simulink model "five_bar_model_w_g"  (R2018a)
settings: Solver=ode4  StartTime=0.0  StopTime=10.0  FixedStep=1e-4  RelTol=1e-3
values from neighbouring files (symbols this model uses):
  g = -9.80665    [ddyn5.m]    (also in idyn5.m; test_dynamics.m; test_model.m)
  p0 = p(:,1)    [model_parameters_v_1.m]    (also in test_dynamics.m = [x(i);y(i)]; test_kinematics.m = [0; 0.35]; test_model.m = [x0;y0])
  q = [NaN; NaN; NaN; NaN; NaN]    [fkine5.m]    (also in ikine5.m = [q11;q12;q13;q21;q22]; test_model.m = q_mode(:,4))
  q0 = q(:,1)    [model_parameters_v_1.m]    (also in test_dynamics.m = q0(:,4); test_kinematics.m = q0(:,4); test_model.m = q_mode(:,4))
  t0r0 = t0r(:,1)    [model_parameters_v_1.m]    (also in test_model.m = [0;0])
  t0rd0 = t0rd(:,1)    [model_parameters_v_1.m]    (also in test_model.m = [0;0])
  x0 = p(1,1)    [model_parameters_v_1.m]    (also in test_model.m = 0)
  y0 = p(2,1)    [model_parameters_v_1.m]    (also in test_model.m = 0.35)
undefined symbols (not defined in the file or in its folder): X, Y, Z
libraries: sm_lib x25, nesl_utility x7, simulink x1
(part 1 of 2)
settings Model: Creator=jere  LastModifiedBy=jere

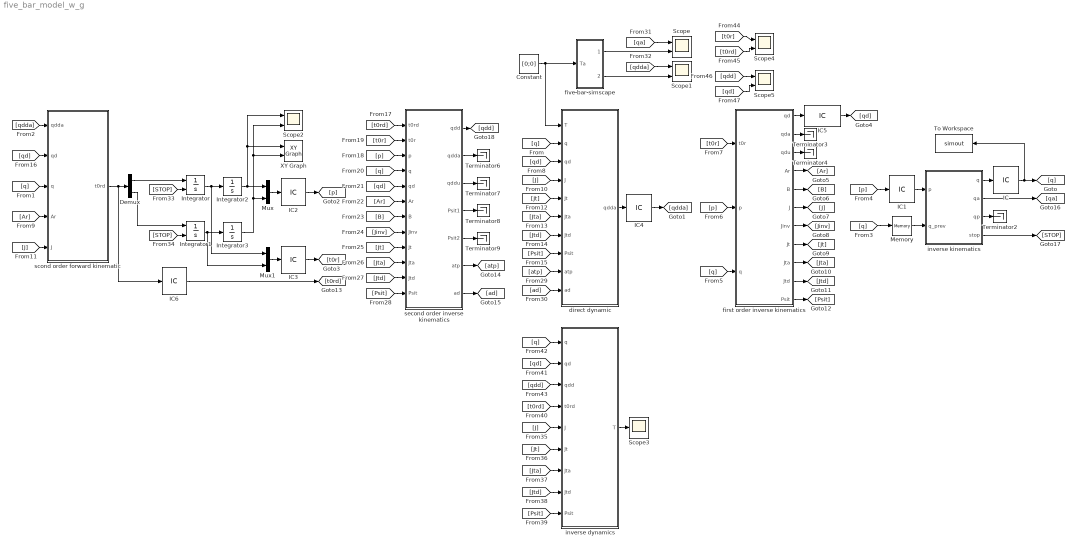
== system five_bar_model_w_g ==
  Constant : Constant  Value=[0;0]
  Demux : Demux  Outputs=2
  IC : InitialCondition  Value=q0
  IC1 : InitialCondition  Value=p0
  IC2 : InitialCondition  Value=p0
  IC3 : InitialCondition  Value=t0r0
  IC4 : InitialCondition  Value=[0;0]
  IC5 : InitialCondition  Value=zeros(5,1)
  IC6 : InitialCondition  Value=t0rd0
  Integrator : Integrator  ExternalReset=level hold
  Integrator1 : Integrator  ExternalReset=level hold
  Integrator2 : Integrator  InitialCondition=x0
  Integrator3 : Integrator  InitialCondition=y0
  Memory : Memory  InitialCondition=q0
  Mux : Mux  Inputs=2
  Mux1 : Mux  Inputs=2
  Scope{,1..2,4..5} (5 alike) : Scope  NumInputPorts=2
  Scope3 : Scope
  Terminator{2..4,6..9} (7 alike) : Terminator
  To Workspace : ToWorkspace  VariableName=simout  SaveFormat=Timeseries  SampleTime=-1
  XY Graph : simulink/Sinks/XY Graph  xmin=-1  xmax=1  ymin=-1  ymax=1  st=-1
  direct dynamic : MATLAB Function  TreatAsAtomicUnit=on
  first order inverse kinematics : MATLAB Function  TreatAsAtomicUnit=on
  five-bar-simscape : Subsystem
  inverse dynamics : MATLAB Function  TreatAsAtomicUnit=on
  inverse kinematics : MATLAB Function  TreatAsAtomicUnit=on
  scond order forward kinematic : MATLAB Function  TreatAsAtomicUnit=on
  second order inverse kinematics : MATLAB Function  TreatAsAtomicUnit=on
  wires:
  Constant/1 -> direct dynamic/1(T), five-bar-simscape/1(Ta)
  five-bar-simscape/2(qdda_o) -> Scope1/2
  [q] -> direct dynamic/2(q)
  [q] -> scond order forward kinematic/3(q)
  IC/1 -> [q], To Workspace/1
  [qdda] -> scond order forward kinematic/1(qdda)
  [q] -> Memory/1
  Memory/1 -> inverse kinematics/2(q_prev)
  inverse kinematics/1(q) -> IC/1
  inverse kinematics/2(qa) -> [qa]
  inverse kinematics/3(qp) -> Terminator2/1
  Integrator/1 -> Integrator2/1, Mux1/1
  Integrator1/1 -> Integrator3/1, Mux1/2
  scond order forward kinematic/1(t0rd) -> Demux/1, IC6/1
  Demux/1 -> Integrator/1
  Demux/2 -> Integrator1/1
  Integrator2/1 -> Scope2/1, XY Graph/1, Mux/1
  Integrator3/1 -> XY Graph/2, Scope2/2, Mux/2
  Mux/1 -> IC2/1
  [p] -> IC1/1
  IC1/1 -> inverse kinematics/1(p)
  [q] -> first order inverse kinematics/3(q)
  [p] -> first order inverse kinematics/2(p)
  [t0r] -> first order inverse kinematics/1(t0r)
  Mux1/1 -> IC3/1
  first order inverse kinematics/1(qd) -> IC5/1
  [qd] -> direct dynamic/3(qd)
  first order inverse kinematics/2(qda) -> Terminator3/1
  first order inverse kinematics/3(qdu) -> Terminator4/1
  first order inverse kinematics/4(Ar) -> [Ar]
  [Ar] -> scond order forward kinematic/4(Ar)
  first order inverse kinematics/5(B) -> [B]
  first order inverse kinematics/6(J) -> [J]
  [J] -> direct dynamic/4(J)
  [J] -> scond order forward kinematic/5(J)
  first order inverse kinematics/7(Jinv) -> [Jinv]
  first order inverse kinematics/8(Jt) -> [Jt]
  [Jt] -> direct dynamic/5(Jt)
  first order inverse kinematics/9(Jta) -> [Jta]
  [Jta] -> direct dynamic/6(Jta)
  first order inverse kinematics/10(Jtd) -> [Jtd]
  [Jtd] -> direct dynamic/7(Jtd)
  first order inverse kinematics/11(Psit) -> [Psit]
  [Psit] -> direct dynamic/8(Psit)
  [qd] -> scond order forward kinematic/2(qd)
  [t0rd] -> second order inverse kinematics/1(t0rd)
  [p] -> second order inverse kinematics/3(p)
  [t0r] -> second order inverse kinematics/2(t0r)
  IC3/1 -> [t0r]
  IC2/1 -> [p]
  [q] -> second order inverse kinematics/4(q)
  [qd] -> second order inverse kinematics/5(qd)
  [Ar] -> second order inverse kinematics/6(Ar)
  [B] -> second order inverse kinematics/7(B)
  [Jinv] -> second order inverse kinematics/8(Jinv)
  [Jt] -> second order inverse kinematics/9(Jt)
  [Jta] -> second order inverse kinematics/10(Jta)
  [Jtd] -> second order inverse kinematics/11(Jtd)
  [Psit] -> second order inverse kinematics/12(Psit)
  second order inverse kinematics/6(atp) -> [atp]
  second order inverse kinematics/7(ad) -> [ad]
  [atp] -> direct dynamic/9(atp)
  [ad] -> direct dynamic/10(ad)
  second order inverse kinematics/1(qdd) -> [qdd]
  second order inverse kinematics/2(qdda) -> Terminator6/1
  second order inverse kinematics/3(qddu) -> Terminator7/1
  second order inverse kinematics/4(Psit1) -> Terminator8/1
  second order inverse kinematics/5(Psit2) -> Terminator9/1
  five-bar-simscape/1(qa_o) -> Scope/2
  direct dynamic/1(qdda) -> IC4/1
  IC5/1 -> [qd]
  [qa] -> Scope/1
  [qdda] -> Scope1/1
  inverse kinematics/4(stop) -> [STOP]
  [STOP] -> Integrator/2
  [STOP] -> Integrator1/2
  inverse dynamics/1(T) -> Scope3/1
  [J] -> inverse dynamics/5(J)
  [Jt] -> inverse dynamics/6(Jt)
  [Jta] -> inverse dynamics/7(Jta)
  [Jtd] -> inverse dynamics/8(Jtd)
  [Psit] -> inverse dynamics/9(Psit)
  [t0rd] -> inverse dynamics/4(t0rd)
  [qd] -> inverse dynamics/2(qd)
  [q] -> inverse dynamics/1(q)
  [qdd] -> inverse dynamics/3(qdd)
  [t0r] -> Scope4/1
  [t0rd] -> Scope4/2
  [qdd] -> Scope5/1
  [qd] -> Scope5/2
  IC4/1 -> [qdda]
  IC6/1 -> [t0rd]

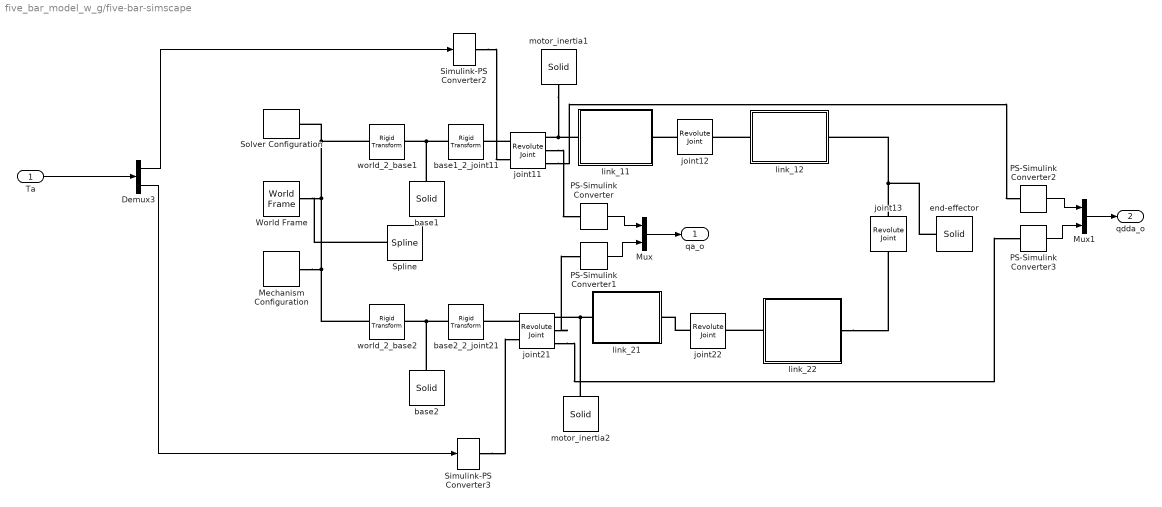
== system five_bar_model_w_g/five-bar-simscape ==
  Ta : Inport
  Demux3 : Demux  Outputs=2
  Mechanism Configuration : sm_lib/Utilities/Mechanism Configuration  UniformGravity=Constant  GravityVector=[0 -9.80665 0]  GravityUnits=m/s^2  LinearizationDelta=0.001
  Mux : Mux  Inputs=2
  Mux1 : Mux  Inputs=2
  PS-Simulink Converter : nesl_utility/PS-Simulink Converter  PhysicalDomain=network_engine_domain  SubClassName=ps_output  LeftPortType=input  RightPortType=output  PseudoPeriodic=off  Frequencies=[]  Unit=rad  AffineConversion=off
  PS-Simulink Converter1 : nesl_utility/PS-Simulink Converter  PhysicalDomain=network_engine_domain  SubClassName=ps_output  LeftPortType=input  RightPortType=output  PseudoPeriodic=off  Frequencies=[]  Unit=rad  AffineConversion=off
  PS-Simulink Converter2 : nesl_utility/PS-Simulink Converter  PhysicalDomain=network_engine_domain  SubClassName=ps_output  LeftPortType=input  RightPortType=output  PseudoPeriodic=off  Frequencies=[]  Unit=1  AffineConversion=off
  PS-Simulink Converter3 : nesl_utility/PS-Simulink Converter  PhysicalDomain=network_engine_domain  SubClassName=ps_output  LeftPortType=input  RightPortType=output  PseudoPeriodic=off  Frequencies=[]  Unit=1  AffineConversion=off
  Simulink-PS Converter2 : nesl_utility/Simulink-PS Converter  PhysicalDomain=network_engine_domain  SubClassName=ps_input  LeftPortType=input  RightPortType=output  PseudoPeriodic=off  Frequencies=[]  NoiseDistribution=none  NoiseParameters=[]  Unit=N*m  AffineConversion=off  FilteringAndDerivatives=provide  SimscapeFilterOrder=1  InputFilterTimeConstant=0.001  UdotUserProvided=0
  Simulink-PS Converter3 : nesl_utility/Simulink-PS Converter  PhysicalDomain=network_engine_domain  SubClassName=ps_input  LeftPortType=input  RightPortType=output  PseudoPeriodic=off  Frequencies=[]  NoiseDistribution=none  NoiseParameters=[]  Unit=N*m  AffineConversion=off  FilteringAndDerivatives=provide  SimscapeFilterOrder=1  InputFilterTimeConstant=0.001  UdotUserProvided=0
  Solver Configuration : nesl_utility/Solver Configuration  PhysicalDomain=network_engine_domain  SubClassName=solver  LeftPortType=input  RightPortType=generic  Tones=[]  Harmonics=[]  SimulateNoise=off  Profile=off  UseLocalSampling=off  EnableSwitchedLinearOptims=on  FrequencyDomain=off  UseCCode=off  RelTol=0.001  AbsTol=1e-06  MinStep=1e-09  ToWorkspace=off  RevertToSquareIcSolve=off  NumHomotopyIterations=100  PhasorMode=off  PhasorModeNumHarmonics=1  DoDC=off  ResidualTolerance=1e-09  UseLocalSolver=off  LocalSolverChoice=NE_BACKWARD_EULER_ADVANCER  LocalSolverSampleTime=0.001  DoFixedCost=off  MaxNonlinIter=3  MaxModeIter=2  LinearAlgebra=Sparse  EquationFormulation=NE_TIME_EF  DelaysMemoryBudget=1024  AutomaticFiltering=on  FilteringTimeConstant=0.001
  Spline : sm_lib/Curves and Surfaces/Spline  DataPoints=[-0.1 0.3; 0.1 0.3]  DataPointsUnits=m  EndConditionType=Natural  GraphicType=FromGeometry  MarkerShape=Sphere  MarkerSize=10  GraphicVisPropType=SimpleVisualProperties  GraphicDiffuseColor=[0 0 0]  GraphicSpecularColor=[0.5 0.5 0.5 1.0]  GraphicAmbientColor=[0.15 0.15 0.15 1.0]  GraphicEmissiveColor=[0.0 0.0 0.0 1.0]  GraphicShininess=75  GraphicOpacity=1.0
      settings: SourceProductName=Simscape Multibody
  World Frame : sm_lib/Frames and Transforms/World Frame
  base1 : sm_lib/Body Elements/Solid  InertiaType=PointMass  Mass=1.72  MassUnits=kg  CenterOfMass=[0 0 0]  CenterOfMassUnits=m  MomentsOfInertia=[1 1 1]  MomentsOfInertiaUnits=kg*m^2  ProductsOfInertia=[0 0 0]  ProductsOfInertiaUnits=kg*m^2  DensityBased=on  Density=1000  DensityUnits=kg/m^3  DoExposeReferenceFrame=on  SerializedFrames=<Frames/>  GraphicType=FromGeometry  MarkerShape=Sphere  MarkerSize=10  GraphicVisPropType=SimpleVisualProperties  GraphicDiffuseColor=[1.0 1.0 0.0]  GraphicSpecularColor=[0.5 0.5 0.5 1.0]  GraphicAmbientColor=[0.15 0.15 0.15 1.0]  GraphicEmissiveColor=[0.0 0.0 0.0 1.0]  GraphicShininess=75  GraphicOpacity=1.0  GeometryShape=FromFile  RectangleSize=[1 1]  RectangleSizeUnits=m  BrickDimensions=[1 1 1]  BrickDimensionUnits=m  CylinderRadius=1  CylinderRadiusUnits=m  CylinderLength=1  CylinderLengthUnits=m  SphereRadius=1  SphereRadiusUnits=m  EllipsoidRadii=[1 1 1]  EllipsoidRadiiUnits=m  ExtrusionCrossSection=[1 1; -1 1; -1 -1; 1 -1]  ExtrusionCrossSectionUnits=m  ExtrusionLength=1  ExtrusionLengthUnits=m  PolygonNumSides=3  PolygonOuterRadius=1  PolygonOuterRadiusUnits=m  ExtGeomFileType=STL  ExtGeomFileName=/home/jere/Documentos/simulacionPF/5-bar-model/meshes/nema23_75mm_8mm.stl  ExtGeomFileUnits=mm  RevolutionCrossSection=[1 1; 1 -1; 2 -1; 2 1]  RevolutionCrossSectionUnits=m  RevolutionExtent=Full  RevolutionAngle=180  RevolutionAngleUnits=deg
  base1_2_joint11 : sm_lib/Frames and Transforms/Rigid Transform  TranslationMethod=Cartesian  TranslationStandardOffset=0  TranslationLengthUnit=mm  TranslationStandardAxis=+Z  TranslationCartesianOffset=[0 0 2]  TranslationROffset=0  TranslationROffsetUnits=m  TranslationZOffset=0  TranslationZOffsetUnits=m  TranslationThetaOffset=0  TranslationThetaOffsetUnits=deg  RotationMethod=None  RotationAngleUnits=deg  RotationStandardAxis=+Z  RotationAngle=0.0  RotationArbitraryAxis=[0 0 1]  FollAlignAxisA=+X  BaseAlignAxisA=+Y  FollAlignAxisB=+Y  BaseAlignAxisB=+Z  RotationSequenceAxes=FollowerAxes  RotationSequence=XYX  RotationSequenceAngles=[0 0 0]  RotationSequenceAnglesUnits=deg  RotationMatrix=[1 0 0; 0 1 0; 0 0 1]
  base2 : sm_lib/Body Elements/Solid  InertiaType=PointMass  Mass=1.72  MassUnits=kg  CenterOfMass=[0 0 0]  CenterOfMassUnits=m  MomentsOfInertia=[1 1 1]  MomentsOfInertiaUnits=kg*m^2  ProductsOfInertia=[0 0 0]  ProductsOfInertiaUnits=kg*m^2  DensityBased=on  Density=1000  DensityUnits=kg/m^3  DoExposeReferenceFrame=on  SerializedFrames=<Frames/>  GraphicType=FromGeometry  MarkerShape=Sphere  MarkerSize=10  GraphicVisPropType=SimpleVisualProperties  GraphicDiffuseColor=[1.0 1.0 0.0]  GraphicSpecularColor=[0.5 0.5 0.5 1.0]  GraphicAmbientColor=[0.15 0.15 0.15 1.0]  GraphicEmissiveColor=[0.0 0.0 0.0 1.0]  GraphicShininess=75  GraphicOpacity=1.0  GeometryShape=FromFile  RectangleSize=[1 1]  RectangleSizeUnits=m  BrickDimensions=[1 1 1]  BrickDimensionUnits=m  CylinderRadius=1  CylinderRadiusUnits=m  CylinderLength=1  CylinderLengthUnits=m  SphereRadius=1  SphereRadiusUnits=m  EllipsoidRadii=[1 1 1]  EllipsoidRadiiUnits=m  ExtrusionCrossSection=[1 1; -1 1; -1 -1; 1 -1]  ExtrusionCrossSectionUnits=m  ExtrusionLength=1  ExtrusionLengthUnits=m  PolygonNumSides=3  PolygonOuterRadius=1  PolygonOuterRadiusUnits=m  ExtGeomFileType=STL  ExtGeomFileName=/home/jere/Documentos/simulacionPF/5-bar-model/meshes/nema23_75mm_8mm.stl  ExtGeomFileUnits=mm  RevolutionCrossSection=[1 1; 1 -1; 2 -1; 2 1]  RevolutionCrossSectionUnits=m  RevolutionExtent=Full  RevolutionAngle=180  RevolutionAngleUnits=deg
  base2_2_joint21 : sm_lib/Frames and Transforms/Rigid Transform  TranslationMethod=Cartesian  TranslationStandardOffset=0  TranslationLengthUnit=mm  TranslationStandardAxis=+Z  TranslationCartesianOffset=[0 0 2]  TranslationROffset=0  TranslationROffsetUnits=m  TranslationZOffset=0  TranslationZOffsetUnits=m  TranslationThetaOffset=0  TranslationThetaOffsetUnits=deg  RotationMethod=None  RotationAngleUnits=deg  RotationStandardAxis=+Z  RotationAngle=0.0  RotationArbitraryAxis=[0 0 1]  FollAlignAxisA=+X  BaseAlignAxisA=+Y  FollAlignAxisB=+Y  BaseAlignAxisB=+Z  RotationSequenceAxes=FollowerAxes  RotationSequence=XYX  RotationSequenceAngles=[0 0 0]  RotationSequenceAnglesUnits=deg  RotationMatrix=[1 0 0; 0 1 0; 0 0 1]
  end-effector : sm_lib/Body Elements/Solid  InertiaType=PointMass  Mass=0.272  MassUnits=kg  CenterOfMass=[0 0 0]  CenterOfMassUnits=m  MomentsOfInertia=[1 1 1]  MomentsOfInertiaUnits=kg*m^2  ProductsOfInertia=[0 0 0]  ProductsOfInertiaUnits=kg*m^2  DensityBased=on  Density=1000  DensityUnits=kg/m^3  DoExposeReferenceFrame=on  SerializedFrames=<Frames/>  GraphicType=FromGeometry  MarkerShape=Sphere  MarkerSize=10  GraphicVisPropType=SimpleVisualProperties  GraphicDiffuseColor=[1.0 1.0 0.0]  GraphicSpecularColor=[0.5 0.5 0.5 1.0]  GraphicAmbientColor=[0.15 0.15 0.15 1.0]  GraphicEmissiveColor=[0.0 0.0 0.0 1.0]  GraphicShininess=75  GraphicOpacity=1.0  GeometryShape=Sphere  RectangleSize=[1 1]  RectangleSizeUnits=m  BrickDimensions=[1 1 1]  BrickDimensionUnits=m  CylinderRadius=1  CylinderRadiusUnits=m  CylinderLength=1  CylinderLengthUnits=m  SphereRadius=1  SphereRadiusUnits=mm  EllipsoidRadii=[1 1 1]  EllipsoidRadiiUnits=m  ExtrusionCrossSection=[1 1; -1 1; -1 -1; 1 -1]  ExtrusionCrossSectionUnits=m  ExtrusionLength=1  ExtrusionLengthUnits=m  PolygonNumSides=3  PolygonOuterRadius=1  PolygonOuterRadiusUnits=m  ExtGeomFileType=STL  ExtGeomFileName=D:\PartsMechanism\propiedades\nema23_75mm_8mm.stl  ExtGeomFileUnits=mm  RevolutionCrossSection=[1 1; 1 -1; 2 -1; 2 1]  RevolutionCrossSectionUnits=m  RevolutionExtent=Full  RevolutionAngle=180  RevolutionAngleUnits=deg
  joint11 : sm_lib/Joints/Revolute Joint  SenseConstraintForce=off  SenseConstraintForceX=off  SenseConstraintForceY=off  SenseConstraintForceZ=off  SenseConstraintTorque=off  SenseConstraintTorqueX=off  SenseConstraintTorqueY=off  SenseConstraintTorqueZ=off  SenseTotalForce=off  SenseTotalForceX=off  SenseTotalForceY=off  SenseTotalForceZ=off  SenseTotalTorque=off  SenseTotalTorqueX=off  SenseTotalTorqueY=off  SenseTotalTorqueZ=off  CompositeWrenchDir=FollowerOnBase  CompositeWrenchFrame=BaseFrame  EquilibriumPosition=0  EquilibriumPositionUnits=rad  SpringStiffness=0  SpringStiffnessUnits=N*m/deg  DampingCoefficient=1.5e-1  DampingCoefficientUnits=N*m/(rad/s)  TorqueActuationMode=InputTorque  MotionActuationMode=ComputedMotion  SensePosition=on  SenseVelocity=off  SenseAcceleration=on  SenseTorqueForce=off  PositionTargetSpecify=on  PositionTargetPriority=High  PositionTargetValue=q(1,1)  PositionTargetValueUnits=rad  VelocityTargetSpecify=off  VelocityTargetPriority=High  VelocityTargetValue=1  VelocityTargetValueUnits=rad/s
  joint12 : sm_lib/Joints/Revolute Joint  SenseConstraintForce=off  SenseConstraintForceX=off  SenseConstraintForceY=off  SenseConstraintForceZ=off  SenseConstraintTorque=off  SenseConstraintTorqueX=off  SenseConstraintTorqueY=off  SenseConstraintTorqueZ=off  SenseTotalForce=off  SenseTotalForceX=off  SenseTotalForceY=off  SenseTotalForceZ=off  SenseTotalTorque=off  SenseTotalTorqueX=off  SenseTotalTorqueY=off  SenseTotalTorqueZ=off  CompositeWrenchDir=FollowerOnBase  CompositeWrenchFrame=BaseFrame  EquilibriumPosition=0  EquilibriumPositionUnits=rad  SpringStiffness=0  SpringStiffnessUnits=N*m/deg  DampingCoefficient=0  DampingCoefficientUnits=N*m/(rad/s)  TorqueActuationMode=NoTorque  MotionActuationMode=ComputedMotion  SensePosition=off  SenseVelocity=off  SenseAcceleration=off  SenseTorqueForce=off  PositionTargetSpecify=off  PositionTargetPriority=High  PositionTargetValue=q(2,1)  PositionTargetValueUnits=rad  VelocityTargetSpecify=off  VelocityTargetPriority=High  VelocityTargetValue=100  VelocityTargetValueUnits=rad/s
  joint13 : sm_lib/Joints/Revolute Joint  SenseConstraintForce=off  SenseConstraintForceX=off  SenseConstraintForceY=off  SenseConstraintForceZ=off  SenseConstraintTorque=off  SenseConstraintTorqueX=off  SenseConstraintTorqueY=off  SenseConstraintTorqueZ=off  SenseTotalForce=off  SenseTotalForceX=off  SenseTotalForceY=off  SenseTotalForceZ=off  SenseTotalTorque=off  SenseTotalTorqueX=off  SenseTotalTorqueY=off  SenseTotalTorqueZ=off  CompositeWrenchDir=FollowerOnBase  CompositeWrenchFrame=BaseFrame  EquilibriumPosition=0  EquilibriumPositionUnits=rad  SpringStiffness=0  SpringStiffnessUnits=N*m/deg  DampingCoefficient=0  DampingCoefficientUnits=N*m/(rad/s)  TorqueActuationMode=NoTorque  MotionActuationMode=ComputedMotion  SensePosition=off  SenseVelocity=off  SenseAcceleration=off  SenseTorqueForce=off  PositionTargetSpecify=off  PositionTargetPriority=High  PositionTargetValue=270  PositionTargetValueUnits=rad  VelocityTargetSpecify=off  VelocityTargetPriority=High  VelocityTargetValue=100  VelocityTargetValueUnits=rad/s
  joint21 : sm_lib/Joints/Revolute Joint  SenseConstraintForce=off  SenseConstraintForceX=off  SenseConstraintForceY=off  SenseConstraintForceZ=off  SenseConstraintTorque=off  SenseConstraintTorqueX=off  SenseConstraintTorqueY=off  SenseConstraintTorqueZ=off  SenseTotalForce=off  SenseTotalForceX=off  SenseTotalForceY=off  SenseTotalForceZ=off  SenseTotalTorque=off  SenseTotalTorqueX=off  SenseTotalTorqueY=off  SenseTotalTorqueZ=off  CompositeWrenchDir=FollowerOnBase  CompositeWrenchFrame=BaseFrame  EquilibriumPosition=0  EquilibriumPositionUnits=rad  SpringStiffness=0  SpringStiffnessUnits=N*m/deg  DampingCoefficient=1.5e-1  DampingCoefficientUnits=N*m/(rad/s)  TorqueActuationMode=InputTorque  MotionActuationMode=ComputedMotion  SensePosition=on  SenseVelocity=off  SenseAcceleration=on  SenseTorqueForce=off  PositionTargetSpecify=on  PositionTargetPriority=High  PositionTargetValue=q(4,1)  PositionTargetValueUnits=rad  VelocityTargetSpecify=off  VelocityTargetPriority=High  VelocityTargetValue=100  VelocityTargetValueUnits=rad/s
  joint22 : sm_lib/Joints/Revolute Joint  SenseConstraintForce=off  SenseConstraintForceX=off  SenseConstraintForceY=off  SenseConstraintForceZ=off  SenseConstraintTorque=off  SenseConstraintTorqueX=off  SenseConstraintTorqueY=off  SenseConstraintTorqueZ=off  SenseTotalForce=off  SenseTotalForceX=off  SenseTotalForceY=off  SenseTotalForceZ=off  SenseTotalTorque=off  SenseTotalTorqueX=off  SenseTotalTorqueY=off  SenseTotalTorqueZ=off  CompositeWrenchDir=FollowerOnBase  CompositeWrenchFrame=BaseFrame  EquilibriumPosition=0  EquilibriumPositionUnits=rad  SpringStiffness=0  SpringStiffnessUnits=N*m/deg  DampingCoefficient=0  DampingCoefficientUnits=N*m/(rad/s)  TorqueActuationMode=NoTorque  MotionActuationMode=ComputedMotion  SensePosition=off  SenseVelocity=off  SenseAcceleration=off  SenseTorqueForce=off  PositionTargetSpecify=off  PositionTargetPriority=High  PositionTargetValue=q(5,1)  PositionTargetValueUnits=rad  VelocityTargetSpecify=off  VelocityTargetPriority=High  VelocityTargetValue=100  VelocityTargetValueUnits=rad/s
  link_11 : Subsystem
  link_12 : Subsystem
  link_21 : Subsystem
  link_22 : Subsystem
  motor_inertia1 : sm_lib/Body Elements/Solid  InertiaType=Custom  Mass=0  MassUnits=kg  CenterOfMass=[0 0 0]  CenterOfMassUnits=m  MomentsOfInertia="[0  0 4.8e-5]"  MomentsOfInertiaUnits=kg*m^2  ProductsOfInertia=[0 0 0]  ProductsOfInertiaUnits=kg*m^2  DensityBased=on  Density=1000  DensityUnits=kg/m^3  DoExposeReferenceFrame=on  SerializedFrames=<Frames/>  GraphicType=FromGeometry  MarkerShape=Sphere  MarkerSize=10  GraphicVisPropType=SimpleVisualProperties  GraphicDiffuseColor=[1.0 1.0 0.0]  GraphicSpecularColor=[0.5 0.5 0.5 1.0]  GraphicAmbientColor=[0.15 0.15 0.15 1.0]  GraphicEmissiveColor=[0.0 0.0 0.0 1.0]  GraphicShininess=75  GraphicOpacity=1.0  GeometryShape=Sphere  RectangleSize=[1 1]  RectangleSizeUnits=m  BrickDimensions=[1 1 1]  BrickDimensionUnits=m  CylinderRadius=1  CylinderRadiusUnits=m  CylinderLength=1  CylinderLengthUnits=m  SphereRadius=1  SphereRadiusUnits=mm  EllipsoidRadii=[1 1 1]  EllipsoidRadiiUnits=m  ExtrusionCrossSection=[1 1; -1 1; -1 -1; 1 -1]  ExtrusionCrossSectionUnits=m  ExtrusionLength=1  ExtrusionLengthUnits=m  PolygonNumSides=3  PolygonOuterRadius=1  PolygonOuterRadiusUnits=m  ExtGeomFileType=STL  ExtGeomFileName=D:\PartsMechanism\propiedades\nema23_75mm_8mm.stl  ExtGeomFileUnits=mm  RevolutionCrossSection=[1 1; 1 -1; 2 -1; 2 1]  RevolutionCrossSectionUnits=m  RevolutionExtent=Full  RevolutionAngle=180  RevolutionAngleUnits=deg
  motor_inertia2 : sm_lib/Body Elements/Solid  InertiaType=Custom  Mass=0  MassUnits=kg  CenterOfMass=[0 0 0]  CenterOfMassUnits=m  MomentsOfInertia=[0 0 4.8e-5]  MomentsOfInertiaUnits=kg*m^2  ProductsOfInertia=[0 0 0]  ProductsOfInertiaUnits=kg*m^2  DensityBased=on  Density=1000  DensityUnits=kg/m^3  DoExposeReferenceFrame=on  SerializedFrames=<Frames/>  GraphicType=FromGeometry  MarkerShape=Sphere  MarkerSize=10  GraphicVisPropType=SimpleVisualProperties  GraphicDiffuseColor=[1.0 1.0 0.0]  GraphicSpecularColor=[0.5 0.5 0.5 1.0]  GraphicAmbientColor=[0.15 0.15 0.15 1.0]  GraphicEmissiveColor=[0.0 0.0 0.0 1.0]  GraphicShininess=75  GraphicOpacity=1.0  GeometryShape=Sphere  RectangleSize=[1 1]  RectangleSizeUnits=m  BrickDimensions=[1 1 1]  BrickDimensionUnits=m  CylinderRadius=1  CylinderRadiusUnits=m  CylinderLength=1  CylinderLengthUnits=m  SphereRadius=1  SphereRadiusUnits=mm  EllipsoidRadii=[1 1 1]  EllipsoidRadiiUnits=m  ExtrusionCrossSection=[1 1; -1 1; -1 -1; 1 -1]  ExtrusionCrossSectionUnits=m  ExtrusionLength=1  ExtrusionLengthUnits=m  PolygonNumSides=3  PolygonOuterRadius=1  PolygonOuterRadiusUnits=m  ExtGeomFileType=STL  ExtGeomFileName=D:\PartsMechanism\propiedades\nema23_75mm_8mm.stl  ExtGeomFileUnits=mm  RevolutionCrossSection=[1 1; 1 -1; 2 -1; 2 1]  RevolutionCrossSectionUnits=m  RevolutionExtent=Full  RevolutionAngle=180  RevolutionAngleUnits=deg
  world_2_base1 : sm_lib/Frames and Transforms/Rigid Transform  TranslationMethod=Cartesian  TranslationStandardOffset=0  TranslationLengthUnit=mm  TranslationStandardAxis=+Z  TranslationCartesianOffset=[-125 0 0]  TranslationROffset=0  TranslationROffsetUnits=m  TranslationZOffset=0  TranslationZOffsetUnits=m  TranslationThetaOffset=0  TranslationThetaOffsetUnits=deg  RotationMethod=None  RotationAngleUnits=deg  RotationStandardAxis=+Z  RotationAngle=0.0  RotationArbitraryAxis=[0 0 1]  FollAlignAxisA=+X  BaseAlignAxisA=+Y  FollAlignAxisB=+Y  BaseAlignAxisB=+Z  RotationSequenceAxes=FollowerAxes  RotationSequence=XYX  RotationSequenceAngles=[0 0 0]  RotationSequenceAnglesUnits=deg  RotationMatrix=[1 0 0; 0 1 0; 0 0 1]
  world_2_base2 : sm_lib/Frames and Transforms/Rigid Transform  TranslationMethod=Cartesian  TranslationStandardOffset=0  TranslationLengthUnit=mm  TranslationStandardAxis=+Z  TranslationCartesianOffset=[125 0 0]  TranslationROffset=0  TranslationROffsetUnits=m  TranslationZOffset=0  TranslationZOffsetUnits=m  TranslationThetaOffset=0  TranslationThetaOffsetUnits=deg  RotationMethod=None  RotationAngleUnits=deg  RotationStandardAxis=+Z  RotationAngle=0.0  RotationArbitraryAxis=[0 0 1]  FollAlignAxisA=+X  BaseAlignAxisA=+Y  FollAlignAxisB=+Y  BaseAlignAxisB=+Z  RotationSequenceAxes=FollowerAxes  RotationSequence=XYX  RotationSequenceAngles=[0 0 0]  RotationSequenceAnglesUnits=deg  RotationMatrix=[1 0 0; 0 1 0; 0 0 1]
  qa_o : Outport
  qdda_o : Outport  Port=2
  wires:
  PS-Simulink Converter/1 -> Mux/1
  PS-Simulink Converter3/1 -> Mux1/2
  PS-Simulink Converter1/1 -> Mux/2
  PS-Simulink Converter2/1 -> Mux1/1
  Mux/1 -> qa_o/1
  Mux1/1 -> qdda_o/1
  Ta/1 -> Demux3/1
  Demux3/1 -> Simulink-PS Converter2/1
  Demux3/2 -> Simulink-PS Converter3/1
  connections:
  joint12/LConn1 -- link_11/RConn1
  joint22/LConn1 -- link_21/RConn1
  world_2_base2/LConn1 -- Mechanism Configuration/RConn1 -- Spline/LConn1 -- World Frame/RConn1 -- world_2_base1/LConn1 -- Solver Configuration/RConn1
  link_21/LConn1 -- joint21/RConn1 -- motor_inertia2/RConn1
  base1/RConn1 -- base1_2_joint11/LConn1 -- world_2_base1/RConn1
  base2_2_joint21/LConn1 -- base2/RConn1 -- world_2_base2/RConn1
  joint11/LConn1 -- base1_2_joint11/RConn1
  link_11/LConn1 -- motor_inertia1/RConn1 -- joint11/RConn1
  joint21/LConn1 -- base2_2_joint21/RConn1
  joint13/LConn1 -- end-effector/RConn1 -- link_12/RConn1
  link_22/RConn1 -- joint13/RConn1
  link_22/LConn1 -- joint22/RConn1
  link_12/LConn1 -- joint12/RConn1
  joint11/RConn2 -- PS-Simulink Converter/LConn1
  joint21/RConn2 -- PS-Simulink Converter1/LConn1
  joint21/RConn3 -- PS-Simulink Converter3/LConn1
  joint11/RConn3 -- PS-Simulink Converter2/LConn1
  Simulink-PS Converter2/RConn1 -- joint11/LConn2
  Simulink-PS Converter3/RConn1 -- joint21/LConn2

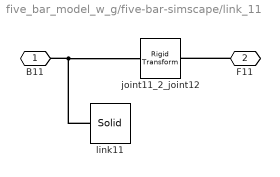
== system five_bar_model_w_g/five-bar-simscape/link_11 ==
  joint11_2_joint12 : sm_lib/Frames and Transforms/Rigid Transform  TranslationMethod=Cartesian  TranslationStandardOffset=0  TranslationLengthUnit=mm  TranslationStandardAxis=+Z  TranslationCartesianOffset=[205 -3 20]  TranslationROffset=0  TranslationROffsetUnits=m  TranslationZOffset=0  TranslationZOffsetUnits=m  TranslationThetaOffset=0  TranslationThetaOffsetUnits=deg  RotationMethod=None  RotationAngleUnits=deg  RotationStandardAxis=+Z  RotationAngle=0.0  RotationArbitraryAxis=[0 0 1]  FollAlignAxisA=+X  BaseAlignAxisA=+Y  FollAlignAxisB=+Y  BaseAlignAxisB=+Z  RotationSequenceAxes=FollowerAxes  RotationSequence=XYX  RotationSequenceAngles=[0 0 0]  RotationSequenceAnglesUnits=deg  RotationMatrix=[1 0 0; 0 1 0; 0 0 1]
  link11 : sm_lib/Body Elements/Solid  InertiaType=Custom  Mass=83.731  MassUnits=g  CenterOfMass=[1.44 8.82 1.19]  CenterOfMassUnits=cm  MomentsOfInertia=[5653.251 63.763 5693.528]  MomentsOfInertiaUnits=g*cm^2  ProductsOfInertia=[0 0 0]  ProductsOfInertiaUnits=g*cm^2  DensityBased=on  Density=1000  DensityUnits=kg/m^3  DoExposeReferenceFrame=off  SerializedFrames=<Frames><Frame><Id>Frame1</Id><Value><Name>F1</Name><Origin><Source>ReferenceFrame</Source><FeatureName></FeatureName></Origin><PrimaryAxis><DefinedDirection>+Z</DefinedDirection><Source>ReferenceFrame</Source><SourceDirection>+Z</SourceDirection><FeatureName></FeatureName></PrimaryAxis><SecondaryAxis><DefinedDirection>+X</DefinedDirection><Source>ReferenceFrame</Source><SourceDirection>+Y</SourceDirection><FeatureName></FeatureName></SecondaryAxis></Value></Frame></Frames>  GraphicType=FromGeometry  MarkerShape=Sphere  MarkerSize=10  GraphicVisPropType=SimpleVisualProperties  GraphicDiffuseColor=[0.0 0.0 0.8]  GraphicSpecularColor=[0.5 0.5 0.5 1.0]  GraphicAmbientColor=[0.15 0.15 0.15 1.0]  GraphicEmissiveColor=[0.0 0.0 0.0 1.0]  GraphicShininess=75  GraphicOpacity=1.0  GeometryShape=FromFile  RectangleSize=[1 1]  RectangleSizeUnits=m  BrickDimensions=[1 1 1]  BrickDimensionUnits=m  CylinderRadius=1  CylinderRadiusUnits=m  CylinderLength=1  CylinderLengthUnits=m  SphereRadius=1  SphereRadiusUnits=m  EllipsoidRadii=[1 1 1]  EllipsoidRadiiUnits=m  ExtrusionCrossSection=[1 1; -1 1; -1 -1; 1 -1]  ExtrusionCrossSectionUnits=m  ExtrusionLength=1  ExtrusionLengthUnits=m  PolygonNumSides=3  PolygonOuterRadius=1  PolygonOuterRadiusUnits=m  ExtGeomFileType=STL  ExtGeomFileName=/home/jere/Documentos/simulacionPF/5-bar-model/meshes/link_11.stl  ExtGeomFileUnits=mm  RevolutionCrossSection=[1 1; 1 -1; 2 -1; 2 1]  RevolutionCrossSectionUnits=m  RevolutionExtent=Full  RevolutionAngle=180  RevolutionAngleUnits=deg
  B11 : PMIOPort  Side=Left
  F11 : PMIOPort  Port=2  Side=Right
  connections:
  F11/RConn1 -- joint11_2_joint12/RConn1
  link11/LConn1 -- B11/RConn1 -- joint11_2_joint12/LConn1

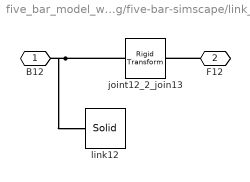
== system five_bar_model_w_g/five-bar-simscape/link_12 ==
  joint12_2_join13 : sm_lib/Frames and Transforms/Rigid Transform  TranslationMethod=Cartesian  TranslationStandardOffset=0  TranslationLengthUnit=mm  TranslationStandardAxis=+Z  TranslationCartesianOffset=[205 0 15]  TranslationROffset=0  TranslationROffsetUnits=m  TranslationZOffset=0  TranslationZOffsetUnits=m  TranslationThetaOffset=0  TranslationThetaOffsetUnits=deg  RotationMethod=None  RotationAngleUnits=deg  RotationStandardAxis=+Z  RotationAngle=0.0  RotationArbitraryAxis=[0 0 1]  FollAlignAxisA=+X  BaseAlignAxisA=+Y  FollAlignAxisB=+Y  BaseAlignAxisB=+Z  RotationSequenceAxes=FollowerAxes  RotationSequence=XYX  RotationSequenceAngles=[0 0 0]  RotationSequenceAnglesUnits=deg  RotationMatrix=[1 0 0; 0 1 0; 0 0 1]
  link12 : sm_lib/Body Elements/Solid  InertiaType=Custom  Mass=72.020  MassUnits=g  CenterOfMass=[-1.24 10.25 0.75]  CenterOfMassUnits=cm  MomentsOfInertia=[4580.984 35.23 4605.847]  MomentsOfInertiaUnits=g*cm^2  ProductsOfInertia=[0 0 0]  ProductsOfInertiaUnits=g*cm^2  DensityBased=on  Density=1000  DensityUnits=kg/m^3  DoExposeReferenceFrame=off  SerializedFrames=<Frames><Frame><Id>Frame1</Id><Value><Name>F1</Name><Origin><Source>ReferenceFrame</Source><FeatureName></FeatureName></Origin><PrimaryAxis><DefinedDirection>+Z</DefinedDirection><Source>ReferenceFrame</Source><SourceDirection>+Z</SourceDirection><FeatureName></FeatureName></PrimaryAxis><SecondaryAxis><DefinedDirection>+X</DefinedDirection><Source>ReferenceFrame</Source><SourceDirection>+Y</SourceDirection><FeatureName></FeatureName></SecondaryAxis></Value></Frame></Frames>  GraphicType=FromGeometry  MarkerShape=Sphere  MarkerSize=10  GraphicVisPropType=SimpleVisualProperties  GraphicDiffuseColor=[0.0 0.8 0.0]  GraphicSpecularColor=[0.5 0.5 0.5 1.0]  GraphicAmbientColor=[0.15 0.15 0.15 1.0]  GraphicEmissiveColor=[0.0 0.0 0.0 1.0]  GraphicShininess=75  GraphicOpacity=1.0  GeometryShape=FromFile  RectangleSize=[1 1]  RectangleSizeUnits=m  BrickDimensions=[1 1 1]  BrickDimensionUnits=m  CylinderRadius=1  CylinderRadiusUnits=m  CylinderLength=1  CylinderLengthUnits=m  SphereRadius=1  SphereRadiusUnits=m  EllipsoidRadii=[1 1 1]  EllipsoidRadiiUnits=m  ExtrusionCrossSection=[1 1; -1 1; -1 -1; 1 -1]  ExtrusionCrossSectionUnits=m  ExtrusionLength=1  ExtrusionLengthUnits=m  PolygonNumSides=3  PolygonOuterRadius=1  PolygonOuterRadiusUnits=m  ExtGeomFileType=STL  ExtGeomFileName=/home/jere/Documentos/simulacionPF/5-bar-model/meshes/link_12.stl  ExtGeomFileUnits=mm  RevolutionCrossSection=[1 1; 1 -1; 2 -1; 2 1]  RevolutionCrossSectionUnits=m  RevolutionExtent=Full  RevolutionAngle=180  RevolutionAngleUnits=deg
  B12 : PMIOPort  Side=Left
  F12 : PMIOPort  Port=2  Side=Right
  connections:
  F12/RConn1 -- joint12_2_join13/RConn1
  B12/RConn1 -- link12/LConn1 -- joint12_2_join13/LConn1

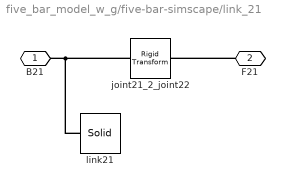
== system five_bar_model_w_g/five-bar-simscape/link_21 ==
  joint21_2_joint22 : sm_lib/Frames and Transforms/Rigid Transform  TranslationMethod=Cartesian  TranslationStandardOffset=0  TranslationLengthUnit=mm  TranslationStandardAxis=+Z  TranslationCartesianOffset=[205 -31 35]  TranslationROffset=0  TranslationROffsetUnits=m  TranslationZOffset=0  TranslationZOffsetUnits=m  TranslationThetaOffset=0  TranslationThetaOffsetUnits=deg  RotationMethod=None  RotationAngleUnits=deg  RotationStandardAxis=+Z  RotationAngle=0  RotationArbitraryAxis=[0 0 1]  FollAlignAxisA=+X  BaseAlignAxisA=+Y  FollAlignAxisB=+Y  BaseAlignAxisB=+Z  RotationSequenceAxes=FollowerAxes  RotationSequence=XYX  RotationSequenceAngles=[0 0 0]  RotationSequenceAnglesUnits=deg  RotationMatrix=[1 0 0; 0 1 0; 0 0 1]
  link21 : sm_lib/Body Elements/Solid  InertiaType=Custom  Mass=102.422  MassUnits=g  CenterOfMass=[1.48 7.21 2.33]  CenterOfMassUnits=cm  MomentsOfInertia=[6910.383 160.537 6923.992]  MomentsOfInertiaUnits=g*cm^2  ProductsOfInertia=[329.041 20.475 275.874]  ProductsOfInertiaUnits=g*cm^2  DensityBased=on  Density=1000  DensityUnits=kg/m^3  DoExposeReferenceFrame=off  SerializedFrames=<Frames><Frame><Id>Frame1</Id><Value><Name>F1</Name><Origin><Source>ReferenceFrame</Source><FeatureName></FeatureName></Origin><PrimaryAxis><DefinedDirection>+Z</DefinedDirection><Source>ReferenceFrame</Source><SourceDirection>+Z</SourceDirection><FeatureName></FeatureName></PrimaryAxis><SecondaryAxis><DefinedDirection>+X</DefinedDirection><Source>ReferenceFrame</Source><SourceDirection>+Y</SourceDirection><FeatureName></FeatureName></SecondaryAxis></Value></Frame></Frames>  GraphicType=FromGeometry  MarkerShape=Sphere  MarkerSize=10  GraphicVisPropType=SimpleVisualProperties  GraphicDiffuseColor=[0.0 0.0 0.8]  GraphicSpecularColor=[0.5 0.5 0.5 1.0]  GraphicAmbientColor=[0.15 0.15 0.15 1.0]  GraphicEmissiveColor=[0.0 0.0 0.0 1.0]  GraphicShininess=75  GraphicOpacity=1.0  GeometryShape=FromFile  RectangleSize=[1 1]  RectangleSizeUnits=m  BrickDimensions=[1 1 1]  BrickDimensionUnits=m  CylinderRadius=1  CylinderRadiusUnits=m  CylinderLength=1  CylinderLengthUnits=m  SphereRadius=1  SphereRadiusUnits=m  EllipsoidRadii=[1 1 1]  EllipsoidRadiiUnits=m  ExtrusionCrossSection=[1 1; -1 1; -1 -1; 1 -1]  ExtrusionCrossSectionUnits=m  ExtrusionLength=1  ExtrusionLengthUnits=m  PolygonNumSides=3  PolygonOuterRadius=1  PolygonOuterRadiusUnits=m  ExtGeomFileType=STL  ExtGeomFileName=/home/jere/Documentos/simulacionPF/5-bar-model/meshes/link_21.stl  ExtGeomFileUnits=mm  RevolutionCrossSection=[1 1; 1 -1; 2 -1; 2 1]  RevolutionCrossSectionUnits=m  RevolutionExtent=Full  RevolutionAngle=180  RevolutionAngleUnits=deg
  B21 : PMIOPort  Side=Left
  F21 : PMIOPort  Port=2  Side=Right
  connections:
  F21/RConn1 -- joint21_2_joint22/RConn1
  link21/LConn1 -- joint21_2_joint22/LConn1 -- B21/RConn1

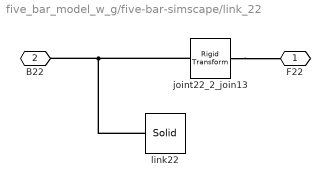
== system five_bar_model_w_g/five-bar-simscape/link_22 ==
  joint22_2_join13 : sm_lib/Frames and Transforms/Rigid Transform  TranslationMethod=Cartesian  TranslationStandardOffset=0  TranslationLengthUnit=mm  TranslationStandardAxis=+Z  TranslationCartesianOffset="[205 0  0]"  TranslationROffset=0  TranslationROffsetUnits=m  TranslationZOffset=0  TranslationZOffsetUnits=m  TranslationThetaOffset=0  TranslationThetaOffsetUnits=deg  RotationMethod=None  RotationAngleUnits=deg  RotationStandardAxis=+Z  RotationAngle=0.0  RotationArbitraryAxis=[0 0 1]  FollAlignAxisA=+X  BaseAlignAxisA=+Y  FollAlignAxisB=+Y  BaseAlignAxisB=+Z  RotationSequenceAxes=FollowerAxes  RotationSequence=XYX  RotationSequenceAngles=[0 0 0]  RotationSequenceAnglesUnits=deg  RotationMatrix=[1 0 0; 0 1 0; 0 0 1]
  link22 : sm_lib/Body Elements/Solid  InertiaType=Custom  Mass=72.020  MassUnits=g  CenterOfMass=[1.24 10.25 0.75]  CenterOfMassUnits=cm  MomentsOfInertia=[4580.628 35.273 4606.029]  MomentsOfInertiaUnits=g*cm^2  ProductsOfInertia=[0 0 0]  ProductsOfInertiaUnits=g*cm^2  DensityBased=on  Density=1000  DensityUnits=kg/m^3  DoExposeReferenceFrame=off  SerializedFrames=<Frames><Frame><Id>Frame1</Id><Value><Name>F1</Name><Origin><Source>ReferenceFrame</Source><FeatureName></FeatureName></Origin><PrimaryAxis><DefinedDirection>+Z</DefinedDirection><Source>ReferenceFrame</Source><SourceDirection>+Z</SourceDirection><FeatureName></FeatureName></PrimaryAxis><SecondaryAxis><DefinedDirection>+X</DefinedDirection><Source>ReferenceFrame</Source><SourceDirection>+Y</SourceDirection><FeatureName></FeatureName></SecondaryAxis></Value></Frame></Frames>  GraphicType=FromGeometry  MarkerShape=Sphere  MarkerSize=10  GraphicVisPropType=SimpleVisualProperties  GraphicDiffuseColor=[0.0 0.8 0.0]  GraphicSpecularColor=[0.5 0.5 0.5 1.0]  GraphicAmbientColor=[0.15 0.15 0.15 1.0]  GraphicEmissiveColor=[0.0 0.0 0.0 1.0]  GraphicShininess=75  GraphicOpacity=1.0  GeometryShape=FromFile  RectangleSize=[1 1]  RectangleSizeUnits=m  BrickDimensions=[1 1 1]  BrickDimensionUnits=m  CylinderRadius=1  CylinderRadiusUnits=m  CylinderLength=1  CylinderLengthUnits=m  SphereRadius=1  SphereRadiusUnits=m  EllipsoidRadii=[1 1 1]  EllipsoidRadiiUnits=m  ExtrusionCrossSection=[1 1; -1 1; -1 -1; 1 -1]  ExtrusionCrossSectionUnits=m  ExtrusionLength=1  ExtrusionLengthUnits=m  PolygonNumSides=3  PolygonOuterRadius=1  PolygonOuterRadiusUnits=m  ExtGeomFileType=STL  ExtGeomFileName=/home/jere/Documentos/simulacionPF/5-bar-model/meshes/link_22.stl  ExtGeomFileUnits=mm  RevolutionCrossSection=[1 1; 1 -1; 2 -1; 2 1]  RevolutionCrossSectionUnits=m  RevolutionExtent=Full  RevolutionAngle=180  RevolutionAngleUnits=deg
  F22 : PMIOPort  Side=Right
  B22 : PMIOPort  Port=2  Side=Left
  connections:
  joint22_2_join13/RConn1 -- F22/RConn1
  link22/LConn1 -- joint22_2_join13/LConn1 -- B22/RConn1

== matlab function five_bar_model_w_g/scond order forward kinematic ==
  data: qdda input; t0rd output; qd input; q input; Ar input; J input
function t0rd  = fsecondkine5(qdda,qd,q,Ar,J)
% This function implement the second-order forward kinematics model of a five bar robot
% @param qdda: active acceleration joints vector 2X1
% @param qd: velocity joints vector 5x1
% @param q: joint positions vector 5x1
% @param Ar: matrix 2x2 for computation of the dynamic model of the PKM
% @param J: kinematic Jacobian matrix of the PKM
% @return t0rd: derivate twist end-effector vector 2X1
    l = 0.205;
    d1 = [-0.125, l, l];
    d2 = [0.125, l, l];
    q1 = q(1:3);
    q2 = q(4:5);
    qd1 = qd(1:3);
    qd2 = qd(4:5);

    wr1 = [cos(q1(1)+q1(2)); sin(q1(1)+q1(2)); 0; 0; 0; 0];
    wr2 = [cos(q2(1)+q2(2)); sin(q2(1)+q2(2)); 0; 0; 0; 0];

    b01a_ = [-d1(2)*qd1(1)*cos(q1(1)) - d1(3)*cos(q1(1)+q1(2))*(qd1(1)+qd1(2));
             -d1(2)*qd1(1)*sin(q1(1)) - d1(3)*sin(q1(1)+q1(2))*(qd1(1)+qd1(2));
             zeros(4,1)];
    b01b_ = [-d1(3)*cos(q1(1)+q1(2));
             -d1(3)*sin(q1(1)+q1(2));
             zeros(4,1)];
    b0p1 = b01a_ * qd1(1) + b01b_ * qd1(2)*(qd1(1)+qd1(2));

    b02a_ = [-d2(2)*qd2(1)*cos(q2(1)) - d2(3)*cos(q2(1)+q2(2))*(qd2(1)+qd2(2));
             -d2(2)*qd2(1)*sin(q2(1)) - d2(3)*sin(q2(1)+q2(2))*(qd2(1)+qd2(2));
             zeros(4,1)];
    b02b_ = [-d2(3)*cos(q2(1)+q2(2));
             -d2(3)*sin(q2(1)+q2(2));
             zeros(4,1)];
    b0p2 = b02a_ * qd2(1) + b02b_ * qd2(2)*(qd2(1)+qd2(2));

    b0p = [(wr1'*b0p1); (wr2'*b0p2)];

    at = pinv(Ar) * b0p;
    t0rd = (J * qdda + at);

== matlab function five_bar_model_w_g/direct dynamic ==
  data: T input; qdda output; q input; qd input; J input; Jt input; Jta input; Jtd input; Psit input; atp input; ad input
function qdda  = ddyn5(T,q,qd,J,Jt,Jta,Jtd,Psit,atp,ad)
    l = 0.205;
    d1 = [-0.125, l, l];
    d2 = [0.125, l, l];
    q1 = q(1:3);
    q2 = q(4:5);
    qd1 = qd(1:3);
    qd2 = qd(4:5);
    % Numerical Solution Dynamics
    % Gravity 
    g = -9.80665;
    
    m11 = 83.731e-3; %kg
    mx11 = m11 * 8.82e-2;
    my11 = 0*m11 * 1.44e-2;
    zz11 = 12375.675e-7;
    
    m21 = 83.731e-3; %kg
    mx21 = m21 * 8.82e-2;
    my21 =  0; %m11 * 1.44e-2;
    zz21 = 12375.675e-7;
%     m21 = 102.422e-3; %kg
%     mx21= m21 * 7.21e-2;
%     my21= m21 * 1.48e-2;
%     zz21 = 12469.254e-7;
    
    m12 = 72.02e-3;
    mx12 = m12 * 10.25e-2;
    my12 = 0*m12 * -1.24e-2;
    zz12 = 12283.918e-7;
    
    m22 = 72.02e-3;
    mx22 = m22 * 10.25e-2;
    my22 = 0*m22 * 1.24e-2;
    zz22 = 12283.918e-7;
    
    %Fricciones fv = viscosa fs= seca
    fv1 = [1.5e-1 0 0];
    fs1 = [1.5e-1 0 0];
    fv2 = [0 0];
    fs2 = [0 0];
    
%     zz11 = 12375.675e-7; % kg-m²
    Ia11 = 0.48 * 0.0001; % kg-m2
    zz11r = zz11 + Ia11 + d1(2)^2 * m12;
%     zz11r = 2.11e-2;

%     zz21 = 12469.254e-7; % kg-m²
    Ia21 = 0.48 * 0.0001; % kg-m2
    zz21r = zz21 + Ia21 + d2(2)^2 * m22;
%     zz21r = 2.24e-2;
    m4 = 0.272;
    % Direct dynamics model
    M11 = zz11r + zz12 + 2 * d1(2) * mx12 * cos(q1(2)) - ...
          2 * d1(2) * my12 * sin(q1(2));

    M12 = zz12 + d1(2) * mx12 * cos(q1(2)) - ...
          d1(2) * my12 * sin(q1(2));
    M21 = M12;

    M44 = zz21r + zz22 + 2 * d2(2) * mx22 * cos(q2(2)) - ...
          2 * d2(2) * my22 * sin(q2(2));

    M45 = zz22 + d2(2) * mx22 * cos(q2(2)) - ...
          d2(2) * my22 * sin(q2(2));
    M54 = M45;

    Mt = [M11 M12  0 0     0;
          M21 zz12 0 0     0;
          0   0    0 0     0;
          0   0    0 M44 M45;
          0   0    0 M54 zz22];

    c1 = -d1(2) * mx12 * qd1(2) * (2 * qd1(1) + qd1(2)) * sin(q1(2)) ...
         -d1(2) * my12 * qd1(2) * (2 * qd1(1) + qd1(2)) * cos(q1(2)) ...
         +fs1(1) * sign(qd1(1)) + fv1(1) * qd1(1) ...
         +(my12*sin(q1(1) + q1(2)) - mx12*cos(q1(1) + q1(2)) ...
         - mx11*cos(q1(1)) + my11*sin(q1(1)) - d1(2)*m12*cos(q1(1)))*g;

    c2 = d1(2) * mx12 * qd1(1)^2 * sin(q1(2)) ...
         +d1(2) * my12 * qd1(1)^2 * cos(q1(2)) ...
         +fs1(2) * sign(qd1(2)) + fv1(2) * qd1(2) ...
         +(my12*sin(q1(1) + q1(2)) - mx12*cos(q1(1) + q1(2)))*g;

    c3 = fs1(3)*sign(qd1(3)) + fv1(3)*qd1(3);

    c4 = -d2(2) * mx22 * qd2(2) * (2 * qd2(1) + qd2(2)) * sin(q2(2)) ...
         -d2(2) * my22 * qd2(2) * (2 * qd2(1) + qd2(2)) * cos(q2(2)) ...
         +fs2(1) * sign( qd2(1) ) + fv2(1) * qd2(1) ...
         +(my22*sin(q2(1) + q2(2)) - mx22*cos(q2(1) + q2(2)) ...
         -mx21*cos(q2(1)) + my21*sin(q2(1)) - d2(2)*m22*cos(q2(1)))*g;

    c5 = d2(2) * mx22 * qd2(1)^2 * sin(q2(2)) ...
         +d2(2) * my22 * qd2(1)^2 * cos(q2(2)) ...
         +fs2(2) * sign(qd2(2)) + fv2(2) * qd2(2) ...
         +(my22*sin(q2(1) + q2(2)) - mx22*cos(q2(1) + q2(2)))*g;

    ct = [c1; c2; c3; c4; c5];

    Et = [1 0 0 0 0;
          0 0 1 0 0;
          0 0 0 1 0;
          0 1 0 0 0;
          0 0 0 0 1];

    M0p = m4 * [eye(2), zeros(2,4); zeros(4,2), zeros(4)];
    % c0p = zeros(6,1); 
    c0p = m4*[0;-g;0;0;0;0]; 
%     J'*Psit'*(c0p)
    % M0r = Psit' * M0p * Psit; % Igual a m4*eye(2)
    M0r = m4 * eye(2);

    Jd = Jtd \ (Jt * J - Jta);

    M = [eye(2), Jd'] * Et'*Mt*Et * [eye(2);Jd] + J'*M0r*J;

    c0r = M0p * atp; % Debe ser igual a 0

    c = [eye(2) Jd'] * Et' * (ct + Mt*Et*[zeros(2,1); ad]) ...
        + J'*Psit'*(c0r+c0p); % if c0r and c0p are 0 the second term is 0

    qdda = pinv(M) * (T-c);

== matlab function five_bar_model_w_g/inverse kinematics ==
  data: p input; q output; q_prev input; qa output; qp output; stop output
function [q,qa,qp,stop] = ikine5(p, q_prev)
% This function implement the inverse kinematic model of a five bar robot
% @parm p: p end-effector coordinate vector 2X1
% @parm q_prev: previos joint position vector 5X1
% @return q: joint positions vector 5x1
% @return qa: active joints positions vector 2X1
% @return qp: underactuated joints positions vector 3X1

    l = 0.205;
    d11 = -0.125;
    d12 = l;
    d13 = l;
    d21 = 0.125;
    d22 = l;
    d23 = l;
    x = p(1);
    y = p(2);
    q_aux = zeros(5,4);

    dist013 = sqrt((p(1)-d11)^2+p(2)^2);
    dist023 = sqrt((p(1)-d21)^2+p(2)^2);
    if dist013 <= 2*l && dist023 <= 2*l
        % q11 = -2*atan((((d11^2 - 2*d11*x - d12^2 + 2*d12*d13 - d13^2 + x^2 + y^2)*(- d11^2 + 2*d11*x + d12^2 + 2*d12*d13 + d13^2 - x^2 - y^2))^(1/2) - 2*d12*y)/(d11^2 - 2*d11*d12 - 2*d11*x + d12^2 + 2*d12*x - d13^2 + x^2 + y^2));
        a1 = -2*d12*(x-d11);
        b1 = -2*d12*y;
        c1 = (x-d11)^2+y^2+d12^2-d13^2;
        q11 = 2*atan((-b1-sqrt(b1^2-c1^2+a1^2)) / (c1-a1));
        if ~isreal(q11)
            q_aux(:,1) = [NaN, NaN, NaN, NaN, NaN]';
            q_aux(:,2) = [NaN, NaN, NaN, NaN, NaN]';
        else
            % q21 = -2*atan((((d21^2 - 2*d21*x - d22^2 + 2*d22*d23 - d23^2 + x^2 + y^2)*(- d21^2 + 2*d21*x + d22^2 + 2*d22*d23 + d23^2 - x^2 - y^2))^(1/2) - 2*d22*y)/(d21^2 - 2*d21*d22 - 2*d21*x + d22^2 + 2*d22*x - d23^2 + x^2 + y^2));
            a2 = -2*d22*(x-d21);
            b2 = -2*d22*y;
            c2 = (x-d21)^2+y^2+d22^2-d23^2;
            q21 = 2*atan((-b2+sqrt(b2^2-c2^2+a2^2)) /(c2-a2));
            if ~isreal(q21)
                q_aux(:,1) = [NaN, NaN, NaN, NaN, NaN]';
            else
                q12 = - q11 + atan2(y - d12*sin(q11), x - d11 - d12*cos(q11));
                q22 = - q21 + atan2(y - d22*sin(q21), x - d21 - d22*cos(q21));
                q13 = q21 - q12 - q11 + q22;
                q_aux(:,1) = [q11, q12, q13, q21, q22]';
            end
            % q21 = 2*atan((((d21^2 - 2*d21*x - d22^2 + 2*d22*d23 - d23^2 + x^2 + y^2)*(- d21^2 + 2*d21*x + d22^2 + 2*d22*d23 + d23^2 - x^2 - y^2))^(1/2) + 2*d22*y)/(d21^2 - 2*d21*d22 - 2*d21*x + d22^2 + 2*d22*x - d23^2 + x^2 + y^2));
            q21 = 2*atan((-b2-sqrt(b2^2-c2^2+a2^2)) /(c2-a2));
            if ~isreal(q21)
                q_aux(:,2) = [NaN, NaN, NaN, NaN, NaN]';
            else
                q12 = - q11 + atan2(y - d12*sin(q11), x - d11 - d12*cos(q11));
                q22 = - q21 + atan2(y - d22*sin(q21), x - d21 - d22*cos(q21));
                q13 = q21 - q12 - q11 + q22;
                q_aux(:,2) = [q11, q12, q13, q21, q22]';
            end
        end

        % q11 = 2*atan((((d11^2 - 2*d11*x - d12^2 + 2*d12*d13 - d13^2 + x^2 + y^2)*(- d11^2 + 2*d11*x + d12^2 + 2*d12*d13 + d13^2 - x^2 - y^2))^(1/2) + 2*d12*y)/(d11^2 - 2*d11*d12 - 2*d11*x + d12^2 + 2*d12*x - d13^2 + x^2 + y^2));
        q11 = 2*atan((-b1+sqrt(b1^2-c1^2+a1^2)) / (c1-a1));
        if ~isreal(q11)
            q_aux(:,3) = [NaN, NaN, NaN, NaN, NaN]';
            q_aux(:,4) = [NaN, NaN, NaN, NaN, NaN]';
        else
            % q21 = -2*atan((((d21^2 - 2*d21*x - d22^2 + 2*d22*d23 - d23^2 + x^2 + y^2)*(- d21^2 + 2*d21*x + d22^2 + 2*d22*d23 + d23^2 - x^2 - y^2))^(1/2) - 2*d22*y)/(d21^2 - 2*d21*d22 - 2*d21*x + d22^2 + 2*d22*x - d23^2 + x^2 + y^2));
            q21 = 2*atan((-b2+sqrt(b2^2-c2^2+a2^2)) /(c2-a2));
            if ~isreal(q21)
                q_aux(:,3) = [NaN, NaN, NaN, NaN, NaN]';
            else
                q12 = - q11 + atan2(y - d12*sin(q11), x - d11 - d12*cos(q11));
                q22 = - q21 + atan2(y - d22*sin(q21), x - d21 - d22*cos(q21));
                q13 = q21 - q12 - q11 + q22;
                q_aux(:,3) = [q11, q12, q13, q21, q22]';
            end
            % q21 = 2*atan((((d21^2 - 2*d21*x - d22^2 + 2*d22*d23 - d23^2 + x^2 + y^2)*(- d21^2 + 2*d21*x + d22^2 + 2*d22*d23 + d23^2 - x^2 - y^2))^(1/2) + 2*d22*y)/(d21^2 - 2*d21*d22 - 2*d21*x + d22^2 + 2*d22*x - d23^2 + x^2 + y^2));
            q21 = 2*atan((-b2-sqrt(b2^2-c2^2+a2^2)) /(c2-a2));
            if ~isreal(q21)
                q_aux(:,4) = [NaN, NaN, NaN, NaN, NaN]';
            else
                q12 = - q11 + atan2(y - d12*sin(q11), x - d11 - d12*cos(q11));
                q22 = - q21 + atan2(y - d22*sin(q21), x - d21 - d22*cos(q21));
                q13 = q21 - q12 - q11 + q22;
                q_aux(:,4) = [q11, q12, q13, q21, q22]';
            end
        end
        % find the correct working mode base in the previous mode
        % qa(:,i) = [q(1,3);q(4,3)]; 
        if nargin < 2
            q = q_aux; %(:,1);
            qa = [q(1,:); q(4,:)];
            qp = [q(2:3,:); q(5,:)];
        else
            distance_between_q = sum(angdiff(q_aux, q_prev * ones(1,4)).^2);
            index = find(distance_between_q == min(distance_between_q));
            q = q_aux(:,index(1));
            qa = [q(1); q(4)];
            qp = [q(2:3); q(5)];
        end
        stop = false;
    else
        disp('ERROR: point out of work space');
%             q = [NaN; NaN; NaN; NaN; NaN];
            q = q_prev;
            stop = true;
            qa = [q(1); q(4)];
            qp = [q(2:3); q(5)];
        % point out of work space
    end
